simulink model "MdXX_SrcTp"  (R2018b)
settings: Solver=FixedStepDiscrete  StartTime=0.0  StopTime=10.0  FixedStep=0.01  RelTol=1e-3
settings Model: Creator=sn2xws  LastModifiedBy=sn2xws
settings DataIOCC: SaveFormat=StructureWithTime
settings OptimizationCC: DefaultParameterBehavior=Inlined  EnhancedBackFolding=on  PassReuseOutputArgsAs=Individual arguments  ZeroExternalMemoryAtStartup=off  ZeroInternalMemoryAtStartup=off  OptimizeBlockOrder=speed  DifferentSizesBufferReuse=on  OptimizationCustomize=off
settings DebuggingCC: ParameterTunabilityLossMsg=error
settings ModelReferenceCC: ModelReferenceNumInstancesAllowed=Single
settings SFSimCC: MATLABDynamicMemAlloc=off
settings RTWCC: SystemTargetFile=autosar.tlc  GenCodeOnly=on  TemplateMakefile=ert_default_tmf  Description=AUTOSAR  GenerateReport=on  IncludeHyperlinkInReport=on  LaunchReport=on  GenerateTraceInfo=on  GenerateTraceReport=on  GenerateTraceReportSl=on  GenerateTraceReportSf=on  GenerateTraceReportEml=on
settings CodeAppCC: ForceParamTrailComments=on  IgnoreCustomStorageClasses=off  OperatorAnnotations=on  SimulinkDataObjDesc=on  SFDataObjDesc=on  InsertBlockDesc=on
settings STFCustomTargetCC: TargetLangStandard=C99 (ISO)  MultiwordLength=256  ParMdlRefBuildCompliant=on  CompOptLevelCompliant=on  IncludeMdlTerminateFcn=off  CombineOutputUpdateFcns=on  SuppressErrorStatus=on  ERTCustomFileBanners=on  SupportNonFinite=off  SupportComplex=off  SupportContinuousTime=off  SupportNonInlinedSFcns=off  RemoveResetFunc=on  MATLABClassNameForMDSCustomization=Simulink.SoftwareTarget.ERTCustomization  AutosarCompliant=on  UseToolchainInfoCompliant=on  LookupTableObjectStructAxisOrder=2,1,3,4,...  LUTObjectStructOrderEvenSpacing=Size,Table,Breakpoints  SystemTargetFile=autosar.tlc
settings ERTTargetCC: TargetLangStandard=C99 (ISO)  ConcurrentExecutionCompliant=off  IncludeMdlTerminateFcn=off  SuppressErrorStatus=on  SupportNonFinite=off  SupportComplex=off  ModelStepFunctionPrototypeControlCompliant=off  CPPClassGenCompliant=off  AutosarCompliant=on  LookupTableObjectStructAxisOrder=2,1,3,4,...  LUTObjectStructOrderEvenSpacing=Size,Table,Breakpoints  InlinedParameterPlacement=NonHierarchical  ERTCustomFileTemplate=example_file_process.tlc

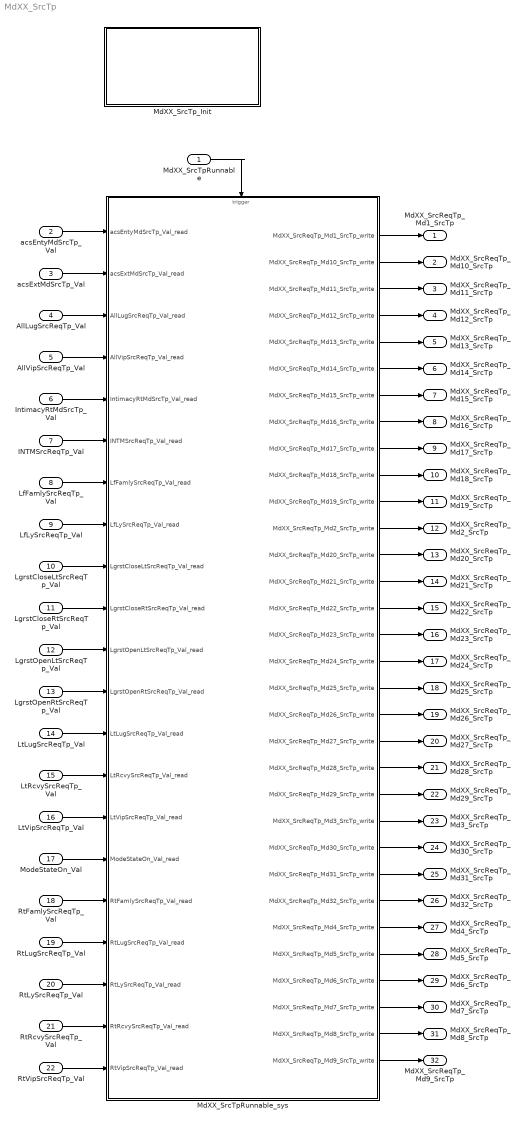
== system MdXX_SrcTp ==
  MdXX_SrcTpRunnable : Inport  SampleTime=0.01  OutputFunctionCall=on
  acsEntyMdSrcTp_Val : Inport  Port=2  OutDataTypeStr=Enum: SrcReqTp1  PortDimensions=1
  acsExtMdSrcTp_Val : Inport  Port=3  OutDataTypeStr=Enum: SrcReqTp1  PortDimensions=1
  AllLugSrcReqTp_Val : Inport  Port=4  OutDataTypeStr=Enum: SrcReqTp1  PortDimensions=1
  AllVipSrcReqTp_Val : Inport  Port=5  OutDataTypeStr=Enum: SrcReqTp1  PortDimensions=1
  IntimacyRtMdSrcTp_Val : Inport  Port=6  OutDataTypeStr=Enum: SrcReqTp1  PortDimensions=1
  INTMSrcReqTp_Val : Inport  Port=7  OutDataTypeStr=Enum: SrcReqTp1  PortDimensions=1
  LfFamlySrcReqTp_Val : Inport  Port=8  OutDataTypeStr=Enum: SrcReqTp1  PortDimensions=1
  LfLySrcReqTp_Val : Inport  Port=9  OutDataTypeStr=Enum: SrcReqTp1  PortDimensions=1
  LgrstCloseLtSrcReqTp_Val : Inport  Port=10  OutDataTypeStr=Enum: SrcReqTp1  PortDimensions=1
  LgrstCloseRtSrcReqTp_Val : Inport  Port=11  OutDataTypeStr=Enum: SrcReqTp1  PortDimensions=1
  LgrstOpenLtSrcReqTp_Val : Inport  Port=12  OutDataTypeStr=Enum: SrcReqTp1  PortDimensions=1
  LgrstOpenRtSrcReqTp_Val : Inport  Port=13  OutDataTypeStr=Enum: SrcReqTp1  PortDimensions=1
  LtLugSrcReqTp_Val : Inport  Port=14  OutDataTypeStr=Enum: SrcReqTp1  PortDimensions=1
  LtRcvySrcReqTp_Val : Inport  Port=15  OutDataTypeStr=Enum: SrcReqTp1  PortDimensions=1
  LtVipSrcReqTp_Val : Inport  Port=16  OutDataTypeStr=Enum: SrcReqTp1  PortDimensions=1
  ModeStateOn_Val : Inport  Port=17  OutDataTypeStr=boolean  PortDimensions=1
  RtFamlySrcReqTp_Val : Inport  Port=18  OutDataTypeStr=Enum: SrcReqTp1  PortDimensions=1
  RtLugSrcReqTp_Val : Inport  Port=19  OutDataTypeStr=Enum: SrcReqTp1  PortDimensions=1
  RtLySrcReqTp_Val : Inport  Port=20  OutDataTypeStr=Enum: SrcReqTp1  PortDimensions=1
  RtRcvySrcReqTp_Val : Inport  Port=21  OutDataTypeStr=Enum: SrcReqTp1  PortDimensions=1
  RtVipSrcReqTp_Val : Inport  Port=22  OutDataTypeStr=Enum: SrcReqTp1  PortDimensions=1
  MdXX_SrcTpRunnable_sys : Subsystem
  MdXX_SrcTp_Init : Subsystem
  MdXX_SrcReqTp_Md1_SrcTp : Outport  OutDataTypeStr=Enum: SrcReqTp1  PortDimensions=1
  MdXX_SrcReqTp_Md10_SrcTp : Outport  Port=2  OutDataTypeStr=Enum: SrcReqTp1  PortDimensions=1
  MdXX_SrcReqTp_Md11_SrcTp : Outport  Port=3  OutDataTypeStr=Enum: SrcReqTp1  PortDimensions=1
  MdXX_SrcReqTp_Md12_SrcTp : Outport  Port=4  OutDataTypeStr=Enum: SrcReqTp1  PortDimensions=1
  MdXX_SrcReqTp_Md13_SrcTp : Outport  Port=5  OutDataTypeStr=Enum: SrcReqTp1  PortDimensions=1
  MdXX_SrcReqTp_Md14_SrcTp : Outport  Port=6  OutDataTypeStr=Enum: SrcReqTp1  PortDimensions=1
  MdXX_SrcReqTp_Md15_SrcTp : Outport  Port=7  OutDataTypeStr=Enum: SrcReqTp1  PortDimensions=1
  MdXX_SrcReqTp_Md16_SrcTp : Outport  Port=8  OutDataTypeStr=Enum: SrcReqTp1  PortDimensions=1
  MdXX_SrcReqTp_Md17_SrcTp : Outport  Port=9  OutDataTypeStr=Enum: SrcReqTp1  PortDimensions=1
  MdXX_SrcReqTp_Md18_SrcTp : Outport  Port=10  OutDataTypeStr=Enum: SrcReqTp1  PortDimensions=1
  MdXX_SrcReqTp_Md19_SrcTp : Outport  Port=11  OutDataTypeStr=Enum: SrcReqTp1  PortDimensions=1
  MdXX_SrcReqTp_Md2_SrcTp : Outport  Port=12  OutDataTypeStr=Enum: SrcReqTp1  PortDimensions=1
  MdXX_SrcReqTp_Md20_SrcTp : Outport  Port=13  OutDataTypeStr=Enum: SrcReqTp1  PortDimensions=1
  MdXX_SrcReqTp_Md21_SrcTp : Outport  Port=14  OutDataTypeStr=Enum: SrcReqTp1  PortDimensions=1
  MdXX_SrcReqTp_Md22_SrcTp : Outport  Port=15  OutDataTypeStr=Enum: SrcReqTp1  PortDimensions=1
  MdXX_SrcReqTp_Md23_SrcTp : Outport  Port=16  OutDataTypeStr=Enum: SrcReqTp1  PortDimensions=1
  MdXX_SrcReqTp_Md24_SrcTp : Outport  Port=17  OutDataTypeStr=Enum: SrcReqTp1  PortDimensions=1
  MdXX_SrcReqTp_Md25_SrcTp : Outport  Port=18  OutDataTypeStr=Enum: SrcReqTp1  PortDimensions=1
  MdXX_SrcReqTp_Md26_SrcTp : Outport  Port=19  OutDataTypeStr=Enum: SrcReqTp1  PortDimensions=1
  MdXX_SrcReqTp_Md27_SrcTp : Outport  Port=20  OutDataTypeStr=Enum: SrcReqTp1  PortDimensions=1
  MdXX_SrcReqTp_Md28_SrcTp : Outport  Port=21  OutDataTypeStr=Enum: SrcReqTp1  PortDimensions=1
  MdXX_SrcReqTp_Md29_SrcTp : Outport  Port=22  OutDataTypeStr=Enum: SrcReqTp1  PortDimensions=1
  MdXX_SrcReqTp_Md3_SrcTp : Outport  Port=23  OutDataTypeStr=Enum: SrcReqTp1  PortDimensions=1
  MdXX_SrcReqTp_Md30_SrcTp : Outport  Port=24  OutDataTypeStr=Enum: SrcReqTp1  PortDimensions=1
  MdXX_SrcReqTp_Md31_SrcTp : Outport  Port=25  OutDataTypeStr=Enum: SrcReqTp1  PortDimensions=1
  MdXX_SrcReqTp_Md32_SrcTp : Outport  Port=26  OutDataTypeStr=Enum: SrcReqTp1  PortDimensions=1
  MdXX_SrcReqTp_Md4_SrcTp : Outport  Port=27  OutDataTypeStr=Enum: SrcReqTp1  PortDimensions=1
  MdXX_SrcReqTp_Md5_SrcTp : Outport  Port=28  OutDataTypeStr=Enum: SrcReqTp1  PortDimensions=1
  MdXX_SrcReqTp_Md6_SrcTp : Outport  Port=29  OutDataTypeStr=Enum: SrcReqTp1  PortDimensions=1
  MdXX_SrcReqTp_Md7_SrcTp : Outport  Port=30  OutDataTypeStr=Enum: SrcReqTp1  PortDimensions=1
  MdXX_SrcReqTp_Md8_SrcTp : Outport  Port=31  OutDataTypeStr=Enum: SrcReqTp1  PortDimensions=1
  MdXX_SrcReqTp_Md9_SrcTp : Outport  Port=32  OutDataTypeStr=Enum: SrcReqTp1  PortDimensions=1
  wires:
  acsEntyMdSrcTp_Val/1 -> MdXX_SrcTpRunnable_sys/1(acsEntyMdSrcTp_Val_read)
  acsExtMdSrcTp_Val/1 -> MdXX_SrcTpRunnable_sys/2(acsExtMdSrcTp_Val_read)
  AllLugSrcReqTp_Val/1 -> MdXX_SrcTpRunnable_sys/3(AllLugSrcReqTp_Val_read)
  AllVipSrcReqTp_Val/1 -> MdXX_SrcTpRunnable_sys/4(AllVipSrcReqTp_Val_read)
  IntimacyRtMdSrcTp_Val/1 -> MdXX_SrcTpRunnable_sys/5(IntimacyRtMdSrcTp_Val_read)
  INTMSrcReqTp_Val/1 -> MdXX_SrcTpRunnable_sys/6(INTMSrcReqTp_Val_read)
  LfFamlySrcReqTp_Val/1 -> MdXX_SrcTpRunnable_sys/7(LfFamlySrcReqTp_Val_read)
  LfLySrcReqTp_Val/1 -> MdXX_SrcTpRunnable_sys/8(LfLySrcReqTp_Val_read)
  LgrstCloseLtSrcReqTp_Val/1 -> MdXX_SrcTpRunnable_sys/9(LgrstCloseLtSrcReqTp_Val_read)
  LgrstCloseRtSrcReqTp_Val/1 -> MdXX_SrcTpRunnable_sys/10(LgrstCloseRtSrcReqTp_Val_read)
  LgrstOpenLtSrcReqTp_Val/1 -> MdXX_SrcTpRunnable_sys/11(LgrstOpenLtSrcReqTp_Val_read)
  LgrstOpenRtSrcReqTp_Val/1 -> MdXX_SrcTpRunnable_sys/12(LgrstOpenRtSrcReqTp_Val_read)
  LtLugSrcReqTp_Val/1 -> MdXX_SrcTpRunnable_sys/13(LtLugSrcReqTp_Val_read)
  LtRcvySrcReqTp_Val/1 -> MdXX_SrcTpRunnable_sys/14(LtRcvySrcReqTp_Val_read)
  LtVipSrcReqTp_Val/1 -> MdXX_SrcTpRunnable_sys/15(LtVipSrcReqTp_Val_read)
  ModeStateOn_Val/1 -> MdXX_SrcTpRunnable_sys/16(ModeStateOn_Val_read)
  RtFamlySrcReqTp_Val/1 -> MdXX_SrcTpRunnable_sys/17(RtFamlySrcReqTp_Val_read)
  RtLugSrcReqTp_Val/1 -> MdXX_SrcTpRunnable_sys/18(RtLugSrcReqTp_Val_read)
  RtLySrcReqTp_Val/1 -> MdXX_SrcTpRunnable_sys/19(RtLySrcReqTp_Val_read)
  RtRcvySrcReqTp_Val/1 -> MdXX_SrcTpRunnable_sys/20(RtRcvySrcReqTp_Val_read)
  RtVipSrcReqTp_Val/1 -> MdXX_SrcTpRunnable_sys/21(RtVipSrcReqTp_Val_read)
  MdXX_SrcTpRunnable_sys/1(MdXX_SrcReqTp_Md1_SrcTp_write) -> MdXX_SrcReqTp_Md1_SrcTp/1
  MdXX_SrcTpRunnable_sys/2(MdXX_SrcReqTp_Md10_SrcTp_write) -> MdXX_SrcReqTp_Md10_SrcTp/1
  MdXX_SrcTpRunnable_sys/3(MdXX_SrcReqTp_Md11_SrcTp_write) -> MdXX_SrcReqTp_Md11_SrcTp/1
  MdXX_SrcTpRunnable_sys/4(MdXX_SrcReqTp_Md12_SrcTp_write) -> MdXX_SrcReqTp_Md12_SrcTp/1
  MdXX_SrcTpRunnable_sys/5(MdXX_SrcReqTp_Md13_SrcTp_write) -> MdXX_SrcReqTp_Md13_SrcTp/1
  MdXX_SrcTpRunnable_sys/6(MdXX_SrcReqTp_Md14_SrcTp_write) -> MdXX_SrcReqTp_Md14_SrcTp/1
  MdXX_SrcTpRunnable_sys/7(MdXX_SrcReqTp_Md15_SrcTp_write) -> MdXX_SrcReqTp_Md15_SrcTp/1
  MdXX_SrcTpRunnable_sys/8(MdXX_SrcReqTp_Md16_SrcTp_write) -> MdXX_SrcReqTp_Md16_SrcTp/1
  MdXX_SrcTpRunnable_sys/9(MdXX_SrcReqTp_Md17_SrcTp_write) -> MdXX_SrcReqTp_Md17_SrcTp/1
  MdXX_SrcTpRunnable_sys/10(MdXX_SrcReqTp_Md18_SrcTp_write) -> MdXX_SrcReqTp_Md18_SrcTp/1
  MdXX_SrcTpRunnable_sys/11(MdXX_SrcReqTp_Md19_SrcTp_write) -> MdXX_SrcReqTp_Md19_SrcTp/1
  MdXX_SrcTpRunnable_sys/12(MdXX_SrcReqTp_Md2_SrcTp_write) -> MdXX_SrcReqTp_Md2_SrcTp/1
  MdXX_SrcTpRunnable_sys/13(MdXX_SrcReqTp_Md20_SrcTp_write) -> MdXX_SrcReqTp_Md20_SrcTp/1
  MdXX_SrcTpRunnable_sys/14(MdXX_SrcReqTp_Md21_SrcTp_write) -> MdXX_SrcReqTp_Md21_SrcTp/1
  MdXX_SrcTpRunnable_sys/15(MdXX_SrcReqTp_Md22_SrcTp_write) -> MdXX_SrcReqTp_Md22_SrcTp/1
  MdXX_SrcTpRunnable_sys/16(MdXX_SrcReqTp_Md23_SrcTp_write) -> MdXX_SrcReqTp_Md23_SrcTp/1
  MdXX_SrcTpRunnable_sys/17(MdXX_SrcReqTp_Md24_SrcTp_write) -> MdXX_SrcReqTp_Md24_SrcTp/1
  MdXX_SrcTpRunnable_sys/18(MdXX_SrcReqTp_Md25_SrcTp_write) -> MdXX_SrcReqTp_Md25_SrcTp/1
  MdXX_SrcTpRunnable_sys/19(MdXX_SrcReqTp_Md26_SrcTp_write) -> MdXX_SrcReqTp_Md26_SrcTp/1
  MdXX_SrcTpRunnable_sys/20(MdXX_SrcReqTp_Md27_SrcTp_write) -> MdXX_SrcReqTp_Md27_SrcTp/1
  MdXX_SrcTpRunnable_sys/21(MdXX_SrcReqTp_Md28_SrcTp_write) -> MdXX_SrcReqTp_Md28_SrcTp/1
  MdXX_SrcTpRunnable_sys/22(MdXX_SrcReqTp_Md29_SrcTp_write) -> MdXX_SrcReqTp_Md29_SrcTp/1
  MdXX_SrcTpRunnable_sys/23(MdXX_SrcReqTp_Md3_SrcTp_write) -> MdXX_SrcReqTp_Md3_SrcTp/1
  MdXX_SrcTpRunnable_sys/24(MdXX_SrcReqTp_Md30_SrcTp_write) -> MdXX_SrcReqTp_Md30_SrcTp/1
  MdXX_SrcTpRunnable_sys/25(MdXX_SrcReqTp_Md31_SrcTp_write) -> MdXX_SrcReqTp_Md31_SrcTp/1
  MdXX_SrcTpRunnable_sys/26(MdXX_SrcReqTp_Md32_SrcTp_write) -> MdXX_SrcReqTp_Md32_SrcTp/1
  MdXX_SrcTpRunnable_sys/27(MdXX_SrcReqTp_Md4_SrcTp_write) -> MdXX_SrcReqTp_Md4_SrcTp/1
  MdXX_SrcTpRunnable_sys/28(MdXX_SrcReqTp_Md5_SrcTp_write) -> MdXX_SrcReqTp_Md5_SrcTp/1
  MdXX_SrcTpRunnable_sys/29(MdXX_SrcReqTp_Md6_SrcTp_write) -> MdXX_SrcReqTp_Md6_SrcTp/1
  MdXX_SrcTpRunnable_sys/30(MdXX_SrcReqTp_Md7_SrcTp_write) -> MdXX_SrcReqTp_Md7_SrcTp/1
  MdXX_SrcTpRunnable_sys/31(MdXX_SrcReqTp_Md8_SrcTp_write) -> MdXX_SrcReqTp_Md8_SrcTp/1
  MdXX_SrcTpRunnable_sys/32(MdXX_SrcReqTp_Md9_SrcTp_write) -> MdXX_SrcReqTp_Md9_SrcTp/1
  MdXX_SrcTpRunnable/1 -> MdXX_SrcTpRunnable_sys/Trigger

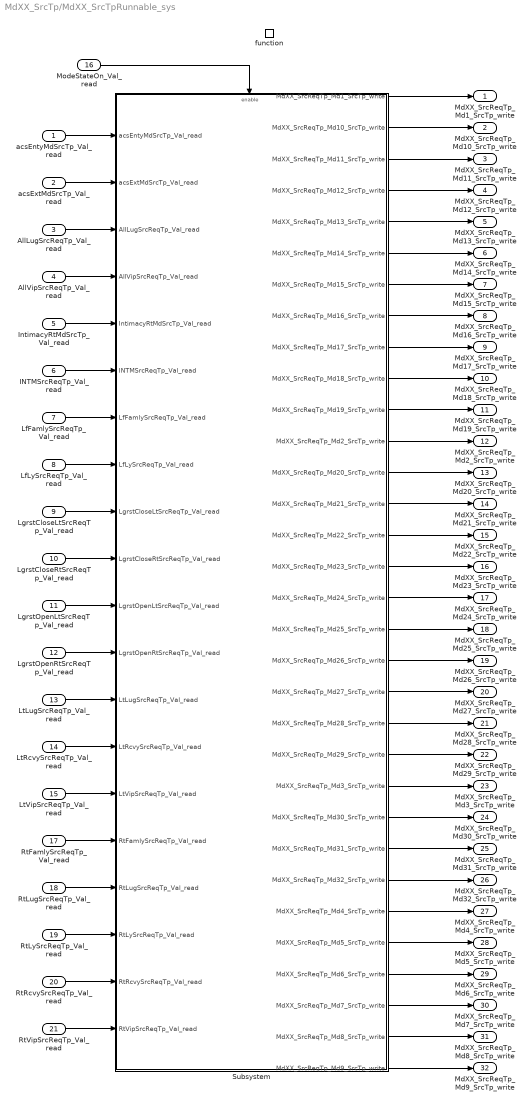
== system MdXX_SrcTp/MdXX_SrcTpRunnable_sys ==
  acsEntyMdSrcTp_Val_read : Inport
  acsExtMdSrcTp_Val_read : Inport  Port=2
  AllLugSrcReqTp_Val_read : Inport  Port=3
  AllVipSrcReqTp_Val_read : Inport  Port=4
  IntimacyRtMdSrcTp_Val_read : Inport  Port=5
  INTMSrcReqTp_Val_read : Inport  Port=6
  LfFamlySrcReqTp_Val_read : Inport  Port=7
  LfLySrcReqTp_Val_read : Inport  Port=8
  LgrstCloseLtSrcReqTp_Val_read : Inport  Port=9
  LgrstCloseRtSrcReqTp_Val_read : Inport  Port=10
  LgrstOpenLtSrcReqTp_Val_read : Inport  Port=11
  LgrstOpenRtSrcReqTp_Val_read : Inport  Port=12
  LtLugSrcReqTp_Val_read : Inport  Port=13
  LtRcvySrcReqTp_Val_read : Inport  Port=14
  LtVipSrcReqTp_Val_read : Inport  Port=15
  ModeStateOn_Val_read : Inport  Port=16
  RtFamlySrcReqTp_Val_read : Inport  Port=17
  RtLugSrcReqTp_Val_read : Inport  Port=18
  RtLySrcReqTp_Val_read : Inport  Port=19
  RtRcvySrcReqTp_Val_read : Inport  Port=20
  RtVipSrcReqTp_Val_read : Inport  Port=21
  function : TriggerPort  TriggerType=function-call  VariantControl=(inherit)  SampleTimeType=periodic  SampleTime=-1
  Subsystem : Subsystem
  MdXX_SrcReqTp_Md1_SrcTp_write : Outport
      settings: EnsureOutportIsVirtual=on
  MdXX_SrcReqTp_Md10_SrcTp_write : Outport  Port=2
      settings: EnsureOutportIsVirtual=on
  MdXX_SrcReqTp_Md11_SrcTp_write : Outport  Port=3
      settings: EnsureOutportIsVirtual=on
  MdXX_SrcReqTp_Md12_SrcTp_write : Outport  Port=4
      settings: EnsureOutportIsVirtual=on
  MdXX_SrcReqTp_Md13_SrcTp_write : Outport  Port=5
      settings: EnsureOutportIsVirtual=on
  MdXX_SrcReqTp_Md14_SrcTp_write : Outport  Port=6
      settings: EnsureOutportIsVirtual=on
  MdXX_SrcReqTp_Md15_SrcTp_write : Outport  Port=7
      settings: EnsureOutportIsVirtual=on
  MdXX_SrcReqTp_Md16_SrcTp_write : Outport  Port=8
      settings: EnsureOutportIsVirtual=on
  MdXX_SrcReqTp_Md17_SrcTp_write : Outport  Port=9
      settings: EnsureOutportIsVirtual=on
  MdXX_SrcReqTp_Md18_SrcTp_write : Outport  Port=10
      settings: EnsureOutportIsVirtual=on
  MdXX_SrcReqTp_Md19_SrcTp_write : Outport  Port=11
      settings: EnsureOutportIsVirtual=on
  MdXX_SrcReqTp_Md2_SrcTp_write : Outport  Port=12
      settings: EnsureOutportIsVirtual=on
  MdXX_SrcReqTp_Md20_SrcTp_write : Outport  Port=13
      settings: EnsureOutportIsVirtual=on
  MdXX_SrcReqTp_Md21_SrcTp_write : Outport  Port=14
      settings: EnsureOutportIsVirtual=on
  MdXX_SrcReqTp_Md22_SrcTp_write : Outport  Port=15
      settings: EnsureOutportIsVirtual=on
  MdXX_SrcReqTp_Md23_SrcTp_write : Outport  Port=16
      settings: EnsureOutportIsVirtual=on
  MdXX_SrcReqTp_Md24_SrcTp_write : Outport  Port=17
      settings: EnsureOutportIsVirtual=on
  MdXX_SrcReqTp_Md25_SrcTp_write : Outport  Port=18
      settings: EnsureOutportIsVirtual=on
  MdXX_SrcReqTp_Md26_SrcTp_write : Outport  Port=19
      settings: EnsureOutportIsVirtual=on
  MdXX_SrcReqTp_Md27_SrcTp_write : Outport  Port=20
      settings: EnsureOutportIsVirtual=on
  MdXX_SrcReqTp_Md28_SrcTp_write : Outport  Port=21
      settings: EnsureOutportIsVirtual=on
  MdXX_SrcReqTp_Md29_SrcTp_write : Outport  Port=22
      settings: EnsureOutportIsVirtual=on
  MdXX_SrcReqTp_Md3_SrcTp_write : Outport  Port=23
      settings: EnsureOutportIsVirtual=on
  MdXX_SrcReqTp_Md30_SrcTp_write : Outport  Port=24
      settings: EnsureOutportIsVirtual=on
  MdXX_SrcReqTp_Md31_SrcTp_write : Outport  Port=25
      settings: EnsureOutportIsVirtual=on
  MdXX_SrcReqTp_Md32_SrcTp_write : Outport  Port=26
      settings: EnsureOutportIsVirtual=on
  MdXX_SrcReqTp_Md4_SrcTp_write : Outport  Port=27
      settings: EnsureOutportIsVirtual=on
  MdXX_SrcReqTp_Md5_SrcTp_write : Outport  Port=28
      settings: EnsureOutportIsVirtual=on
  MdXX_SrcReqTp_Md6_SrcTp_write : Outport  Port=29
      settings: EnsureOutportIsVirtual=on
  MdXX_SrcReqTp_Md7_SrcTp_write : Outport  Port=30
      settings: EnsureOutportIsVirtual=on
  MdXX_SrcReqTp_Md8_SrcTp_write : Outport  Port=31
      settings: EnsureOutportIsVirtual=on
  MdXX_SrcReqTp_Md9_SrcTp_write : Outport  Port=32
      settings: EnsureOutportIsVirtual=on
  wires:
  ModeStateOn_Val_read/1 -> Subsystem/Enable
  acsEntyMdSrcTp_Val_read/1 -> Subsystem/1(acsEntyMdSrcTp_Val_read)
  acsExtMdSrcTp_Val_read/1 -> Subsystem/2(acsExtMdSrcTp_Val_read)
  AllLugSrcReqTp_Val_read/1 -> Subsystem/3(AllLugSrcReqTp_Val_read)
  AllVipSrcReqTp_Val_read/1 -> Subsystem/4(AllVipSrcReqTp_Val_read)
  IntimacyRtMdSrcTp_Val_read/1 -> Subsystem/5(IntimacyRtMdSrcTp_Val_read)
  INTMSrcReqTp_Val_read/1 -> Subsystem/6(INTMSrcReqTp_Val_read)
  LfFamlySrcReqTp_Val_read/1 -> Subsystem/7(LfFamlySrcReqTp_Val_read)
  LfLySrcReqTp_Val_read/1 -> Subsystem/8(LfLySrcReqTp_Val_read)
  LgrstCloseLtSrcReqTp_Val_read/1 -> Subsystem/9(LgrstCloseLtSrcReqTp_Val_read)
  LgrstCloseRtSrcReqTp_Val_read/1 -> Subsystem/10(LgrstCloseRtSrcReqTp_Val_read)
  LgrstOpenLtSrcReqTp_Val_read/1 -> Subsystem/11(LgrstOpenLtSrcReqTp_Val_read)
  LgrstOpenRtSrcReqTp_Val_read/1 -> Subsystem/12(LgrstOpenRtSrcReqTp_Val_read)
  LtLugSrcReqTp_Val_read/1 -> Subsystem/13(LtLugSrcReqTp_Val_read)
  LtRcvySrcReqTp_Val_read/1 -> Subsystem/14(LtRcvySrcReqTp_Val_read)
  LtVipSrcReqTp_Val_read/1 -> Subsystem/15(LtVipSrcReqTp_Val_read)
  RtFamlySrcReqTp_Val_read/1 -> Subsystem/16(RtFamlySrcReqTp_Val_read)
  RtLugSrcReqTp_Val_read/1 -> Subsystem/17(RtLugSrcReqTp_Val_read)
  RtLySrcReqTp_Val_read/1 -> Subsystem/18(RtLySrcReqTp_Val_read)
  RtRcvySrcReqTp_Val_read/1 -> Subsystem/19(RtRcvySrcReqTp_Val_read)
  RtVipSrcReqTp_Val_read/1 -> Subsystem/20(RtVipSrcReqTp_Val_read)
  Subsystem/1(MdXX_SrcReqTp_Md1_SrcTp_write) -> MdXX_SrcReqTp_Md1_SrcTp_write/1
  Subsystem/2(MdXX_SrcReqTp_Md10_SrcTp_write) -> MdXX_SrcReqTp_Md10_SrcTp_write/1
  Subsystem/3(MdXX_SrcReqTp_Md11_SrcTp_write) -> MdXX_SrcReqTp_Md11_SrcTp_write/1
  Subsystem/4(MdXX_SrcReqTp_Md12_SrcTp_write) -> MdXX_SrcReqTp_Md12_SrcTp_write/1
  Subsystem/5(MdXX_SrcReqTp_Md13_SrcTp_write) -> MdXX_SrcReqTp_Md13_SrcTp_write/1
  Subsystem/6(MdXX_SrcReqTp_Md14_SrcTp_write) -> MdXX_SrcReqTp_Md14_SrcTp_write/1
  Subsystem/7(MdXX_SrcReqTp_Md15_SrcTp_write) -> MdXX_SrcReqTp_Md15_SrcTp_write/1
  Subsystem/8(MdXX_SrcReqTp_Md16_SrcTp_write) -> MdXX_SrcReqTp_Md16_SrcTp_write/1
  Subsystem/9(MdXX_SrcReqTp_Md17_SrcTp_write) -> MdXX_SrcReqTp_Md17_SrcTp_write/1
  Subsystem/10(MdXX_SrcReqTp_Md18_SrcTp_write) -> MdXX_SrcReqTp_Md18_SrcTp_write/1
  Subsystem/11(MdXX_SrcReqTp_Md19_SrcTp_write) -> MdXX_SrcReqTp_Md19_SrcTp_write/1
  Subsystem/12(MdXX_SrcReqTp_Md2_SrcTp_write) -> MdXX_SrcReqTp_Md2_SrcTp_write/1
  Subsystem/13(MdXX_SrcReqTp_Md20_SrcTp_write) -> MdXX_SrcReqTp_Md20_SrcTp_write/1
  Subsystem/14(MdXX_SrcReqTp_Md21_SrcTp_write) -> MdXX_SrcReqTp_Md21_SrcTp_write/1
  Subsystem/15(MdXX_SrcReqTp_Md22_SrcTp_write) -> MdXX_SrcReqTp_Md22_SrcTp_write/1
  Subsystem/16(MdXX_SrcReqTp_Md23_SrcTp_write) -> MdXX_SrcReqTp_Md23_SrcTp_write/1
  Subsystem/17(MdXX_SrcReqTp_Md24_SrcTp_write) -> MdXX_SrcReqTp_Md24_SrcTp_write/1
  Subsystem/18(MdXX_SrcReqTp_Md25_SrcTp_write) -> MdXX_SrcReqTp_Md25_SrcTp_write/1
  Subsystem/19(MdXX_SrcReqTp_Md26_SrcTp_write) -> MdXX_SrcReqTp_Md26_SrcTp_write/1
  Subsystem/20(MdXX_SrcReqTp_Md27_SrcTp_write) -> MdXX_SrcReqTp_Md27_SrcTp_write/1
  Subsystem/21(MdXX_SrcReqTp_Md28_SrcTp_write) -> MdXX_SrcReqTp_Md28_SrcTp_write/1
  Subsystem/22(MdXX_SrcReqTp_Md29_SrcTp_write) -> MdXX_SrcReqTp_Md29_SrcTp_write/1
  Subsystem/23(MdXX_SrcReqTp_Md3_SrcTp_write) -> MdXX_SrcReqTp_Md3_SrcTp_write/1
  Subsystem/24(MdXX_SrcReqTp_Md30_SrcTp_write) -> MdXX_SrcReqTp_Md30_SrcTp_write/1
  Subsystem/25(MdXX_SrcReqTp_Md31_SrcTp_write) -> MdXX_SrcReqTp_Md31_SrcTp_write/1
  Subsystem/26(MdXX_SrcReqTp_Md32_SrcTp_write) -> MdXX_SrcReqTp_Md32_SrcTp_write/1
  Subsystem/27(MdXX_SrcReqTp_Md4_SrcTp_write) -> MdXX_SrcReqTp_Md4_SrcTp_write/1
  Subsystem/28(MdXX_SrcReqTp_Md5_SrcTp_write) -> MdXX_SrcReqTp_Md5_SrcTp_write/1
  Subsystem/29(MdXX_SrcReqTp_Md6_SrcTp_write) -> MdXX_SrcReqTp_Md6_SrcTp_write/1
  Subsystem/30(MdXX_SrcReqTp_Md7_SrcTp_write) -> MdXX_SrcReqTp_Md7_SrcTp_write/1
  Subsystem/31(MdXX_SrcReqTp_Md8_SrcTp_write) -> MdXX_SrcReqTp_Md8_SrcTp_write/1
  Subsystem/32(MdXX_SrcReqTp_Md9_SrcTp_write) -> MdXX_SrcReqTp_Md9_SrcTp_write/1

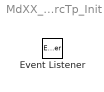
== system MdXX_SrcTp/MdXX_SrcTp_Init ==
  Event Listener : EventListener  EventName=reset

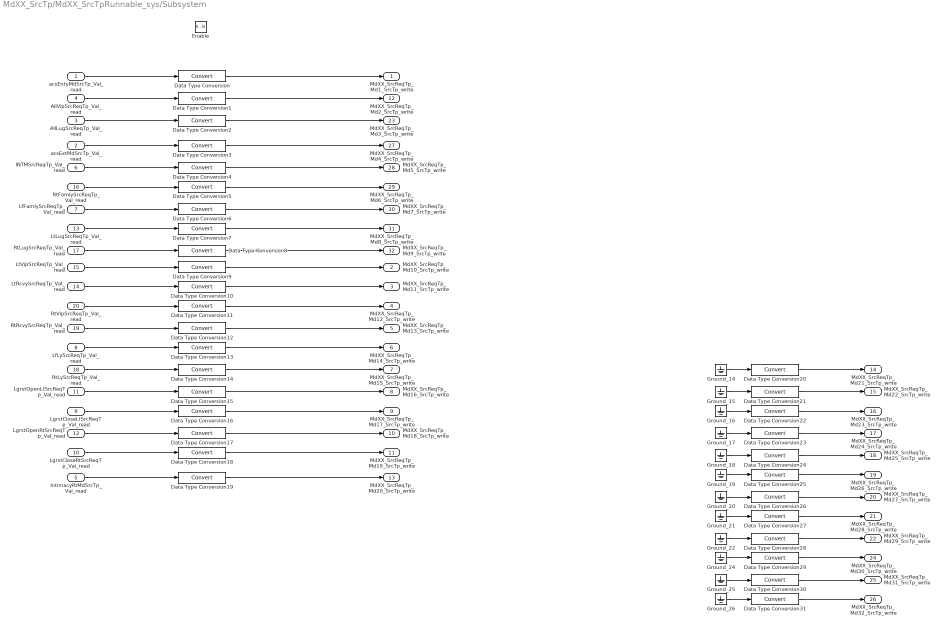
== system MdXX_SrcTp/MdXX_SrcTpRunnable_sys/Subsystem ==
  acsEntyMdSrcTp_Val_read : Inport
  acsExtMdSrcTp_Val_read : Inport  Port=2
  AllLugSrcReqTp_Val_read : Inport  Port=3
  AllVipSrcReqTp_Val_read : Inport  Port=4
  IntimacyRtMdSrcTp_Val_read : Inport  Port=5
  INTMSrcReqTp_Val_read : Inport  Port=6
  LfFamlySrcReqTp_Val_read : Inport  Port=7
  LfLySrcReqTp_Val_read : Inport  Port=8
  LgrstCloseLtSrcReqTp_Val_read : Inport  Port=9
  LgrstCloseRtSrcReqTp_Val_read : Inport  Port=10
  LgrstOpenLtSrcReqTp_Val_read : Inport  Port=11
  LgrstOpenRtSrcReqTp_Val_read : Inport  Port=12
  LtLugSrcReqTp_Val_read : Inport  Port=13
  LtRcvySrcReqTp_Val_read : Inport  Port=14
  LtVipSrcReqTp_Val_read : Inport  Port=15
  RtFamlySrcReqTp_Val_read : Inport  Port=16
  RtLugSrcReqTp_Val_read : Inport  Port=17
  RtLySrcReqTp_Val_read : Inport  Port=18
  RtRcvySrcReqTp_Val_read : Inport  Port=19
  RtVipSrcReqTp_Val_read : Inport  Port=20
  Enable : EnablePort  StatesWhenEnabling=reset
  Data Type Conversion{,1..31} (32 alike) : DataTypeConversion
  Ground_{14..22,24..26} (12 alike) : Ground
  MdXX_SrcReqTp_Md1_SrcTp_write : Outport
  MdXX_SrcReqTp_Md10_SrcTp_write : Outport  Port=2
  MdXX_SrcReqTp_Md11_SrcTp_write : Outport  Port=3
  MdXX_SrcReqTp_Md12_SrcTp_write : Outport  Port=4
  MdXX_SrcReqTp_Md13_SrcTp_write : Outport  Port=5
  MdXX_SrcReqTp_Md14_SrcTp_write : Outport  Port=6
  MdXX_SrcReqTp_Md15_SrcTp_write : Outport  Port=7
  MdXX_SrcReqTp_Md16_SrcTp_write : Outport  Port=8
  MdXX_SrcReqTp_Md17_SrcTp_write : Outport  Port=9
  MdXX_SrcReqTp_Md18_SrcTp_write : Outport  Port=10
  MdXX_SrcReqTp_Md19_SrcTp_write : Outport  Port=11
  MdXX_SrcReqTp_Md2_SrcTp_write : Outport  Port=12
  MdXX_SrcReqTp_Md20_SrcTp_write : Outport  Port=13
  MdXX_SrcReqTp_Md21_SrcTp_write : Outport  Port=14
  MdXX_SrcReqTp_Md22_SrcTp_write : Outport  Port=15
  MdXX_SrcReqTp_Md23_SrcTp_write : Outport  Port=16
  MdXX_SrcReqTp_Md24_SrcTp_write : Outport  Port=17
  MdXX_SrcReqTp_Md25_SrcTp_write : Outport  Port=18
  MdXX_SrcReqTp_Md26_SrcTp_write : Outport  Port=19
  MdXX_SrcReqTp_Md27_SrcTp_write : Outport  Port=20
  MdXX_SrcReqTp_Md28_SrcTp_write : Outport  Port=21
  MdXX_SrcReqTp_Md29_SrcTp_write : Outport  Port=22
  MdXX_SrcReqTp_Md3_SrcTp_write : Outport  Port=23
  MdXX_SrcReqTp_Md30_SrcTp_write : Outport  Port=24
  MdXX_SrcReqTp_Md31_SrcTp_write : Outport  Port=25
  MdXX_SrcReqTp_Md32_SrcTp_write : Outport  Port=26
  MdXX_SrcReqTp_Md4_SrcTp_write : Outport  Port=27
  MdXX_SrcReqTp_Md5_SrcTp_write : Outport  Port=28
  MdXX_SrcReqTp_Md6_SrcTp_write : Outport  Port=29
  MdXX_SrcReqTp_Md7_SrcTp_write : Outport  Port=30
  MdXX_SrcReqTp_Md8_SrcTp_write : Outport  Port=31
  MdXX_SrcReqTp_Md9_SrcTp_write : Outport  Port=32
  wires:
  INTMSrcReqTp_Val_read/1 -> Data Type Conversion4/1
  RtFamlySrcReqTp_Val_read/1 -> Data Type Conversion5/1
  LfFamlySrcReqTp_Val_read/1 -> Data Type Conversion6/1
  AllVipSrcReqTp_Val_read/1 -> Data Type Conversion1/1
  acsEntyMdSrcTp_Val_read/1 -> Data Type Conversion/1
  Ground_25/1 -> Data Type Conversion30/1
  Ground_16/1 -> Data Type Conversion22/1
  Ground_20/1 -> Data Type Conversion26/1
  Ground_18/1 -> Data Type Conversion24/1
  Ground_19/1 -> Data Type Conversion25/1
  Ground_14/1 -> Data Type Conversion20/1
  Ground_15/1 -> Data Type Conversion21/1
  AllLugSrcReqTp_Val_read/1 -> Data Type Conversion2/1
  Ground_22/1 -> Data Type Conversion28/1
  Ground_17/1 -> Data Type Conversion23/1
  Ground_21/1 -> Data Type Conversion27/1
  Ground_24/1 -> Data Type Conversion29/1
  Data Type Conversion19/1 -> MdXX_SrcReqTp_Md20_SrcTp_write/1
  Ground_26/1 -> Data Type Conversion31/1
  Data Type Conversion/1 -> MdXX_SrcReqTp_Md1_SrcTp_write/1
  Data Type Conversion1/1 -> MdXX_SrcReqTp_Md2_SrcTp_write/1
  Data Type Conversion2/1 -> MdXX_SrcReqTp_Md3_SrcTp_write/1
  Data Type Conversion3/1 -> MdXX_SrcReqTp_Md4_SrcTp_write/1
  Data Type Conversion4/1 -> MdXX_SrcReqTp_Md5_SrcTp_write/1
  Data Type Conversion5/1 -> MdXX_SrcReqTp_Md6_SrcTp_write/1
  Data Type Conversion6/1 -> MdXX_SrcReqTp_Md7_SrcTp_write/1
  Data Type Conversion7/1 -> MdXX_SrcReqTp_Md8_SrcTp_write/1
  Data Type Conversion8/1 -> MdXX_SrcReqTp_Md9_SrcTp_write/1
  Data Type Conversion9/1 -> MdXX_SrcReqTp_Md10_SrcTp_write/1
  Data Type Conversion10/1 -> MdXX_SrcReqTp_Md11_SrcTp_write/1
  Data Type Conversion11/1 -> MdXX_SrcReqTp_Md12_SrcTp_write/1
  Data Type Conversion12/1 -> MdXX_SrcReqTp_Md13_SrcTp_write/1
  Data Type Conversion13/1 -> MdXX_SrcReqTp_Md14_SrcTp_write/1
  Data Type Conversion14/1 -> MdXX_SrcReqTp_Md15_SrcTp_write/1
  Data Type Conversion16/1 -> MdXX_SrcReqTp_Md17_SrcTp_write/1
  Data Type Conversion15/1 -> MdXX_SrcReqTp_Md16_SrcTp_write/1
  Data Type Conversion17/1 -> MdXX_SrcReqTp_Md18_SrcTp_write/1
  Data Type Conversion18/1 -> MdXX_SrcReqTp_Md19_SrcTp_write/1
  IntimacyRtMdSrcTp_Val_read/1 -> Data Type Conversion19/1
  LtLugSrcReqTp_Val_read/1 -> Data Type Conversion7/1
  RtLugSrcReqTp_Val_read/1 -> Data Type Conversion8/1
  LfLySrcReqTp_Val_read/1 -> Data Type Conversion13/1
  RtLySrcReqTp_Val_read/1 -> Data Type Conversion14/1
  LgrstOpenLtSrcReqTp_Val_read/1 -> Data Type Conversion15/1
  LgrstCloseLtSrcReqTp_Val_read/1 -> Data Type Conversion16/1
  LgrstOpenRtSrcReqTp_Val_read/1 -> Data Type Conversion17/1
  LgrstCloseRtSrcReqTp_Val_read/1 -> Data Type Conversion18/1
  LtVipSrcReqTp_Val_read/1 -> Data Type Conversion9/1
  LtRcvySrcReqTp_Val_read/1 -> Data Type Conversion10/1
  RtVipSrcReqTp_Val_read/1 -> Data Type Conversion11/1
  RtRcvySrcReqTp_Val_read/1 -> Data Type Conversion12/1
  acsExtMdSrcTp_Val_read/1 -> Data Type Conversion3/1
  Data Type Conversion20/1 -> MdXX_SrcReqTp_Md21_SrcTp_write/1
  Data Type Conversion21/1 -> MdXX_SrcReqTp_Md22_SrcTp_write/1
  Data Type Conversion22/1 -> MdXX_SrcReqTp_Md23_SrcTp_write/1
  Data Type Conversion23/1 -> MdXX_SrcReqTp_Md24_SrcTp_write/1
  Data Type Conversion24/1 -> MdXX_SrcReqTp_Md25_SrcTp_write/1
  Data Type Conversion25/1 -> MdXX_SrcReqTp_Md26_SrcTp_write/1
  Data Type Conversion26/1 -> MdXX_SrcReqTp_Md27_SrcTp_write/1
  Data Type Conversion27/1 -> MdXX_SrcReqTp_Md28_SrcTp_write/1
  Data Type Conversion28/1 -> MdXX_SrcReqTp_Md29_SrcTp_write/1
  Data Type Conversion29/1 -> MdXX_SrcReqTp_Md30_SrcTp_write/1
  Data Type Conversion30/1 -> MdXX_SrcReqTp_Md31_SrcTp_write/1
  Data Type Conversion31/1 -> MdXX_SrcReqTp_Md32_SrcTp_write/1
